simulink model "stace_space_model_final"  (R2020a)
settings: Solver=VariableStepAuto  StartTime=0.0  StopTime=1000  RelTol=1e-3
settings Model: Creator=啊包PC  LastModifiedBy=啊包PC

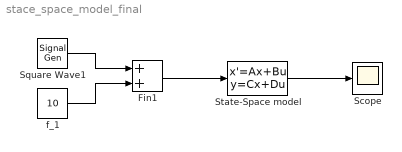
== system stace_space_model_final ==
  Fin1 : Sum
  Scope : Scope
  Square Wave1 : SignalGenerator  WaveForm=square  Amplitude=0.3*10  Frequency=1/60
  State-Space model : StateSpace  A=[-1 1; 1 -7/3]  B=[1/6 ; 1/75]  C=[1 0 ; 0 1]  D=[0 ; 0]  InitialCondition=0
  f_1 : Constant  Value=10
  wires:
  f_1/1 -> Fin1/2
  Square Wave1/1 -> Fin1/1
  State-Space model/1 -> Scope/1
  Fin1/1 -> State-Space model/1
